simulink model "modelePD"  (R2015b)
settings: Solver=VariableStepAuto  StartTime=0.0  StopTime=10.0  RelTol=1e-3
values from neighbouring files (symbols this model uses):
  Beff = 1/80    (= 0.0125)    [commande_robot.m]    (also in sf_loi_avant_RP.m; sf_retour_linearisant_RP.m)
  Jeff = Jm + r^2*m    [commande_robot.m]    (also in sf_loi_avant_RP.m = Jm+r^2*m; sf_retour_linearisant_RP.m = Jm+r^2*m)
  K = (Kd^2)/4    (= 2.25)    [commande_robot.m]
  Kd = 3    [commande_robot.m]
  Km_R = 0.3    [commande_robot.m]    (also in sf_loi_avant_RP.m; sf_retour_linearisant_RP.m)
  r = R(1)    [commande_robot.m]    (also in sf_loi_avant_RP.m; sf_retour_linearisant_RP.m)
libraries: lib_robotRP x4, simulink x2, cstblocks x1
settings Model: Creator=chamand  LastModifiedBy=chamand

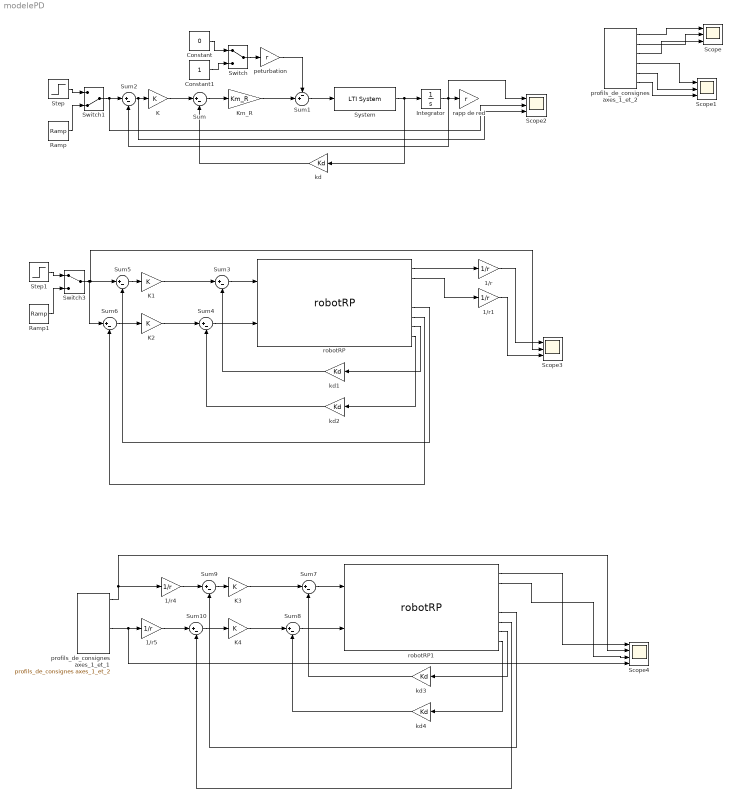
== system modelePD ==
  1/r{,1,4..5} (4 alike) : Gain  Gain=1/r
  Constant : Constant  Value=0
  Constant1 : Constant
  Integrator : Integrator
  K{,1..4} (5 alike) : Gain  Gain=K
  "Km_R " : Gain  Gain=Km_R
  Ramp : simulink/Sources/Ramp  slope=1  start=0  X0=0
  Ramp1 : simulink/Sources/Ramp  slope=1  start=0  X0=0
  Scope{,1..3} (4 alike) : Scope  NumInputPorts=3
  Scope4 : Scope  NumInputPorts=4
  Step : Step  Time=0  SampleTime=0
  Step1 : Step  Time=0  SampleTime=0
  Sum{,2..10} (10 alike) : Sum  Inputs=|+-
  Sum1 : Sum  Inputs=-+|
  Switch : ManualSwitch
  Switch1 : ManualSwitch  CurrentSetting=0
  Switch3 : ManualSwitch
  System : cstblocks/LTI System  sys=tf(1,[Jeff Beff])  IC=[]
  kd{,1..4} (5 alike) : Gain  Gain=Kd
  peturbation : Gain  Gain=r
  profils_de_consignes axes_1_et_1 : lib_robotRP/profils_de_consignes axes_1_et_2
  profils_de_consignes axes_1_et_2 : lib_robotRP/profils_de_consignes axes_1_et_2
  "rapp de red " : Gain  Gain=r
  robotRP : lib_robotRP/robotRP  vecteur_theta_dtheta_initial=[0 ; 1/2/r ; 0 ; 0]  m=15  gX=0  gY=-9.81  F1=0  F2=0  H1=0  H2=0  Km_sur_R=0.3  Jm=0.01  Beff=0.0125  r=1/200
  robotRP1 : lib_robotRP/robotRP  vecteur_theta_dtheta_initial=[0 ; 1/2/r ; 0 ; 0]  m=15  gX=0  gY=-9.81  F1=0  F2=0  H1=0  H2=0  Km_sur_R=0.3  Jm=0.01  Beff=0.0125  r=1/200
  wires:
  profils_de_consignes axes_1_et_2/1 -> Scope/1
  profils_de_consignes axes_1_et_2/2 -> Scope/2
  profils_de_consignes axes_1_et_2/3 -> Scope/3
  profils_de_consignes axes_1_et_2/4 -> Scope1/1
  profils_de_consignes axes_1_et_2/5 -> Scope1/2
  profils_de_consignes axes_1_et_2/6 -> Scope1/3
  K/1 -> Sum/1
  kd/1 -> Sum/2
  Sum/1 -> "Km_R "/1
  System/1 -> kd/1, Integrator/1
  Constant/1 -> Switch/1
  Switch/1 -> peturbation/1
  "Km_R "/1 -> Sum1/2
  peturbation/1 -> Sum1/1
  Sum1/1 -> System/1
  Step/1 -> Switch1/1
  Ramp/1 -> Switch1/2
  Sum2/1 -> Scope2/3, K/1
  Switch1/1 -> Scope2/2, Sum2/1
  Constant1/1 -> Switch/2
  Integrator/1 -> Scope2/1, Sum2/2, "rapp de red "/1
  kd1/1 -> Sum3/2
  Step1/1 -> Switch3/1
  Ramp1/1 -> Switch3/2
  Switch3/1 -> Sum5/1, Scope3/2, Sum6/1
  Sum3/1 -> robotRP/1
  robotRP/7 -> kd1/1
  robotRP/5 -> Sum5/2
  robotRP/1 -> 1/r/1
  1/r/1 -> Scope3/1
  Sum5/1 -> K1/1
  robotRP/2 -> 1/r1/1
  1/r1/1 -> Scope3/3
  robotRP/8 -> kd2/1
  robotRP/6 -> Sum6/2
  Sum6/1 -> K2/1
  kd2/1 -> Sum4/2
  Sum4/1 -> robotRP/2
  K1/1 -> Sum3/1
  K2/1 -> Sum4/1
  kd3/1 -> Sum7/2
  Sum7/1 -> robotRP1/1
  robotRP1/7 -> kd3/1
  robotRP1/5 -> Sum9/2
  robotRP1/1 -> Scope4/1
  Sum9/1 -> K3/1
  robotRP1/2 -> Scope4/3
  robotRP1/8 -> kd4/1
  robotRP1/6 -> Sum10/2
  Sum10/1 -> K4/1
  kd4/1 -> Sum8/2
  Sum8/1 -> robotRP1/2
  K3/1 -> Sum7/1
  K4/1 -> Sum8/1
  profils_de_consignes axes_1_et_1/1 -> Scope4/2, 1/r4/1
  profils_de_consignes axes_1_et_1/4 -> Scope4/4, 1/r5/1
  1/r5/1 -> Sum10/1
  1/r4/1 -> Sum9/1
